simulink model "hw2"  (R2020a)
settings: Solver=VariableStepAuto  StartTime=0.0  StopTime=0.03  RelTol=1e-3
undefined symbols (not defined in the file): alpha, Beq, Bload, Gr, Jeq, Jload, Ke, Kt, La, Ra, Va
settings Model: Creator=helep  LastModifiedBy=JeongHun Hong
settings SFSimCC: CustomCodeUndefinedFunction=UseInterfaceOnly

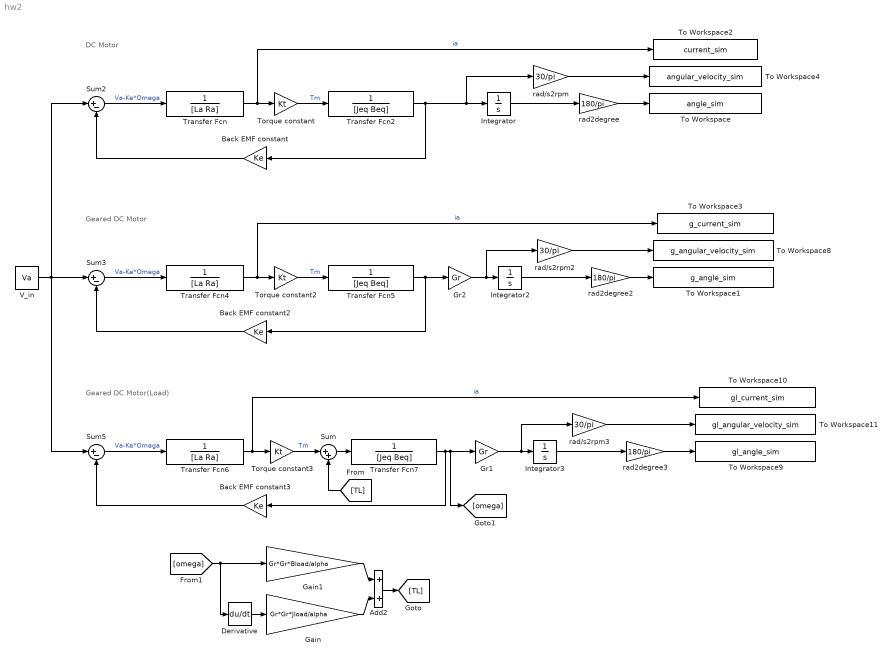
== system hw2 ==
  note: DC Motor
  note: Geared DC Motor
  note: Geared DC Motor(Load)
  Add2 : Sum
  Back EMF constant : Gain  Gain=Ke
  Back EMF constant2 : Gain  Gain=Ke
  Back EMF constant3 : Gain  Gain=Ke
  Derivative : Derivative
  Gain : Gain  Gain=Gr*Gr*Jload/alpha
  Gain1 : Gain  Gain=Gr*Gr*Bload/alpha
  Gr1 : Gain  Gain=Gr
  Gr2 : Gain  Gain=Gr
  Integrator : Integrator
  Integrator2 : Integrator
  Integrator3 : Integrator
  Sum : Sum  Inputs=|++
  Sum2 : Sum  Inputs=|+-
  Sum3 : Sum  Inputs=|+-
  Sum5 : Sum  Inputs=|+-
  To Workspace : ToWorkspace  VariableName=angle_sim  SaveFormat=Structure With Time  SampleTime=-1
  To Workspace1 : ToWorkspace  VariableName=g_angle_sim  SaveFormat=Structure With Time  SampleTime=-1
  To Workspace10 : ToWorkspace  VariableName=gl_current_sim  SaveFormat=Structure With Time  SampleTime=-1
  To Workspace11 : ToWorkspace  VariableName=gl_angular_velocity_sim  SaveFormat=Structure With Time  SampleTime=-1
  To Workspace2 : ToWorkspace  VariableName=current_sim  SaveFormat=Structure With Time  SampleTime=-1
  To Workspace3 : ToWorkspace  VariableName=g_current_sim  SaveFormat=Structure With Time  SampleTime=-1
  To Workspace4 : ToWorkspace  VariableName=angular_velocity_sim  SaveFormat=Structure With Time  SampleTime=-1
  To Workspace8 : ToWorkspace  VariableName=g_angular_velocity_sim  SaveFormat=Structure With Time  SampleTime=-1
  To Workspace9 : ToWorkspace  VariableName=gl_angle_sim  SaveFormat=Structure With Time  SampleTime=-1
  Torque constant : Gain  Gain=Kt
  Torque constant2 : Gain  Gain=Kt
  Torque constant3 : Gain  Gain=Kt
  Transfer Fcn : TransferFcn  Denominator=[La Ra]
  Transfer Fcn2 : TransferFcn  Denominator=[Jeq Beq]
  Transfer Fcn4 : TransferFcn  Denominator=[La Ra]
  Transfer Fcn5 : TransferFcn  Denominator=[Jeq Beq]
  Transfer Fcn6 : TransferFcn  Denominator=[La Ra]
  Transfer Fcn7 : TransferFcn  Denominator=[Jeq Beq]
  V_in : Constant  Value=Va
  rad/s2rpm : Gain  Gain=30/pi
  rad/s2rpm2 : Gain  Gain=30/pi
  rad/s2rpm3 : Gain  Gain=30/pi
  rad2degree : Gain  Gain=180/pi
  rad2degree2 : Gain  Gain=180/pi
  rad2degree3 : Gain  Gain=180/pi
  wires:
  Back EMF constant/1 -> Sum2/2
  Sum2/1 -> Transfer Fcn/1  "Va-Ke*Omega"
  Transfer Fcn/1 -> Torque constant/1, To Workspace2/1  "ia"
  rad2degree/1 -> To Workspace/1
  Integrator/1 -> rad2degree/1
  rad/s2rpm/1 -> To Workspace4/1
  Torque constant/1 -> Transfer Fcn2/1  "Tm"
  Transfer Fcn2/1 -> rad/s2rpm/1, Integrator/1, Back EMF constant/1
  Transfer Fcn5/1 -> Back EMF constant2/1, Gr2/1
  Torque constant2/1 -> Transfer Fcn5/1  "Tm"
  rad/s2rpm2/1 -> To Workspace8/1
  Integrator2/1 -> rad2degree2/1
  Transfer Fcn4/1 -> To Workspace3/1, Torque constant2/1  "ia"
  Sum3/1 -> Transfer Fcn4/1  "Va-Ke*Omega"
  Back EMF constant2/1 -> Sum3/2
  rad2degree2/1 -> To Workspace1/1
  Gr2/1 -> Integrator2/1, rad/s2rpm2/1
  Gr1/1 -> rad/s2rpm3/1, Integrator3/1
  Back EMF constant3/1 -> Sum5/2
  Sum5/1 -> Transfer Fcn6/1  "Va-Ke*Omega"
  V_in/1 -> Sum2/1, Sum5/1, Sum3/1
  Transfer Fcn6/1 -> To Workspace10/1, Torque constant3/1  "ia"
  Integrator3/1 -> rad2degree3/1
  rad/s2rpm3/1 -> To Workspace11/1
  Transfer Fcn7/1 -> Gr1/1, [omega], Back EMF constant3/1
  Torque constant3/1 -> Sum/1  "Tm"
  Sum/1 -> Transfer Fcn7/1
  rad2degree3/1 -> To Workspace9/1
  Derivative/1 -> Gain/1
  [TL] -> Sum/2
  Gain/1 -> Add2/2
  Gain1/1 -> Add2/1
  Add2/1 -> [TL]
  [omega] -> Derivative/1, Gain1/1
